simulink model "WriteRegisterTriggered"  (R2023a)
settings: Solver=FixedStepAuto  StartTime=0.0  StopTime=Inf  FixedStep=SAMPLING_TIME  RelTol=1e-3
undefined symbols (not defined in the file): SAMPLING_TIME
libraries: Interface x3
Description:
  | % Copyright 2023 The MathWorks, Inc.
settings Model: DataDictionary=Parameters.sldd  EnableAccessToBaseWorkspace=off  Creator=sdupertu  LastModifiedBy=sdupertu
settings SolverCC: AlgebraicLoopSolver=TrustRegion
settings OptimizationCC: DefaultParameterBehavior=Inlined  EnhancedBackFolding=on  PassReuseOutputArgsAs=Individual arguments  OptimizeBlockOrder=speed  DifferentSizesBufferReuse=on  OptimizationCustomize=off  EfficientTunableParamExpr=on
settings DebuggingCC: ParameterTunabilityLossMsg=error  UnconnectedInputMsg=warning  UnconnectedOutputMsg=warning  UnconnectedLineMsg=warning  PregeneratedLibrarySubsystemCodeDiagnostic=none  ArithmeticOperatorsInVariantConditions=warning
settings ModelReferenceCC: EnableRefExpFcnMdlSchedulingChecks=on  EnableParallelModelReferenceBuilds=on  SupportModelReferenceSimTargetCustomCode=on
settings SFSimCC: SimCustomHeaderCode="#include \"ParkingMeterMemory.h\""  SimUserSources=ParkingMeterMemory.c  SimUserIncludeDirs=..\Interface_C_files  SimUseLocalCustomCode=off  MATLABDynamicMemAlloc=off  CustomCodeUndefinedFunction=UseInterfaceOnly
settings RTWCC: Description=Embedded Coder  SystemTargetFile=ert.tlc  TemplateMakefile=ert_default_tmf  RTWUseLocalCustomCode=off  RTWUseSimCustomCode=on  CustomHeaderCode="#include \"ParkingMeterMemory.h\""  CustomInclude=..\Interface_C_files  CustomSource=ParkingMeterMemory.c  IncludeHyperlinkInReport=on  DLArmComputeVersion=19.05
settings CodeAppCC: ForceParamTrailComments=on  IgnoreCustomStorageClasses=off  MaxIdLength=61  OperatorAnnotations=on  SimulinkDataObjDesc=on  SFDataObjDesc=on  InsertBlockDesc=on
settings ERTTargetCC: TargetLangStandard=C99 (ISO)  GenerateSampleERTMain=on  InlinedParameterPlacement=NonHierarchical  ERTCustomFileTemplate=example_file_process.tlc

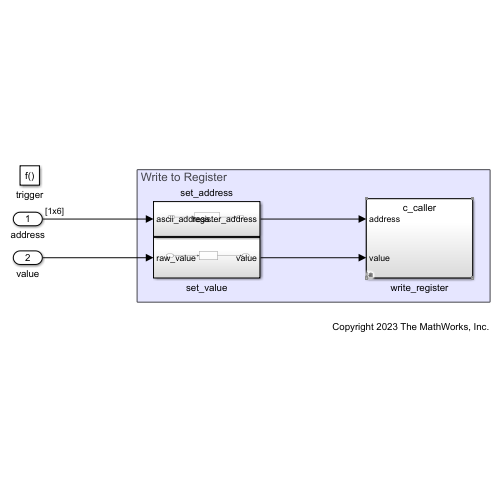
[thumbnail: Simulink's stored preview of the top-level diagram]
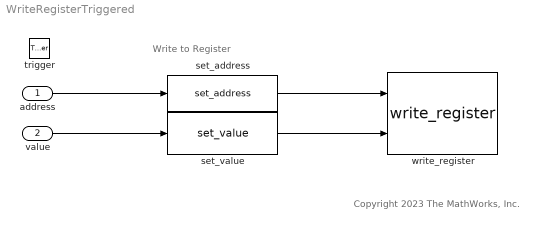
== system WriteRegisterTriggered ==
  note: Copyright 2023 The MathWorks, Inc.
  note: Write to Register
  address : Inport  OutDataTypeStr=uint8  PortDimensions=[1 6]
  value : Inport  Port=2  OutDataTypeStr=uint8  PortDimensions=[1 1]
  trigger : TriggerPort  TriggerType=function-call  VariantControl=Variant  SampleTime=SAMPLING_TIME  PortDimensions=1
  set_address : Interface/set_address  SystemSampleTime=-1  VariantActivationTime=update diagram  Latency=0  AutoFrameSizeCalculation=off
  set_value : Interface/set_value  SystemSampleTime=-1  VariantActivationTime=update diagram  Latency=0  AutoFrameSizeCalculation=off
  write_register : Interface/write_register  SystemSampleTime=-1  VariantControl=Variant1  LabelModeActiveChoice=SRC  VariantActivationTime=update diagram  Latency=0  AutoFrameSizeCalculation=off
  wires:
  set_address/1 -> write_register/1
  value/1 -> set_value/1
  set_value/1 -> write_register/2
  address/1 -> set_address/1
